simulink subsystem "WinchControl"  (R2022b)
settings: Solver=VariableStepAuto  StartTime=0.0  StopTime=10.0  RelTol=1e-3
undefined symbols (not defined in the file): constr, DiscIntNeverNeededParam, params, winchParameter
libraries: simulink x4
settings Model: Creator=dylaneijkelhof  LastModifiedBy=jesse
settings SolverCC: AlgebraicLoopSolver=TrustRegion
settings DebuggingCC: UnconnectedInputMsg=warning  UnconnectedOutputMsg=warning  UnconnectedLineMsg=warning  SFMachineParentedDataDiag=warning
settings ModelReferenceCC: EnableRefExpFcnMdlSchedulingChecks=on

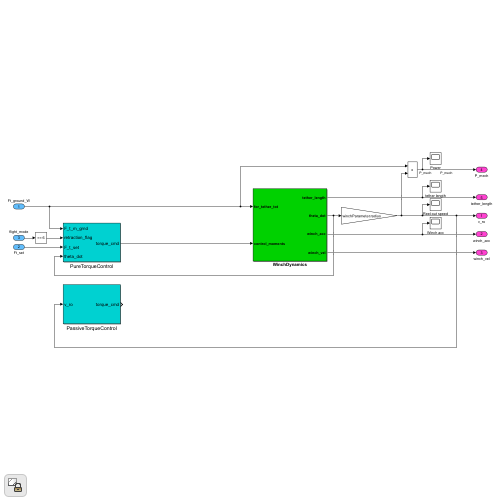
[thumbnail: Simulink's stored preview of the top-level diagram]
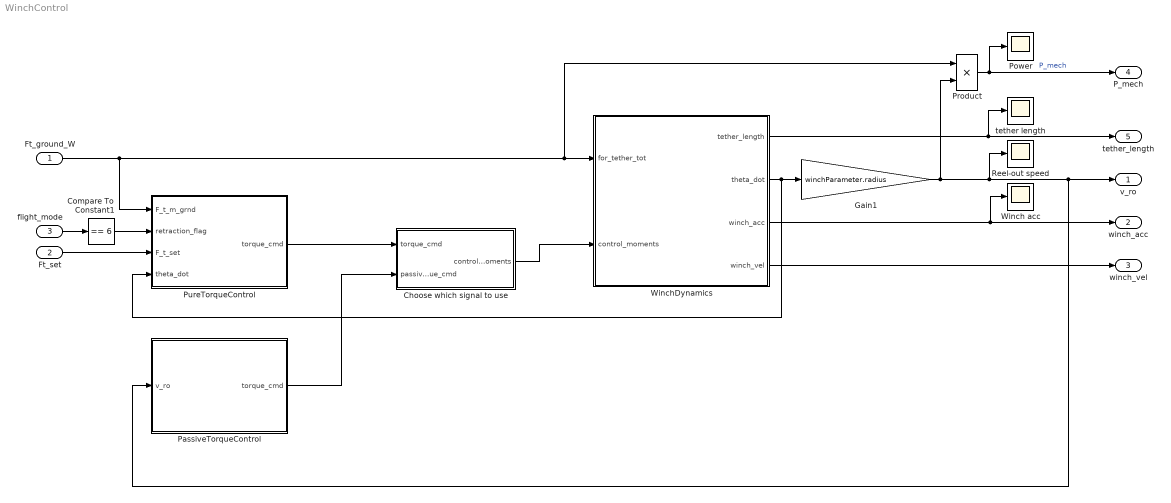
== system WinchControl ==
  Ft_ground_W : Inport  OutDataTypeStr=double  PortDimensions=1
  Ft_set : Inport  Port=2  OutDataTypeStr=double  PortDimensions=1
  flight_mode : Inport  Port=3  OutDataTypeStr=double  PortDimensions=1
  Choose which signal to use : Subsystem
  Compare To Constant1 : simulink/Logic and Bit Operations/Compare To Constant  relop===  const=6  OutDataTypeStr=boolean
  Gain1 : Gain  Gain=winchParameter.radius
  PassiveTorqueControl : Subsystem
  Power : Scope
  Product : Product
  PureTorqueControl : Subsystem
  Reel-out speed : Scope
  Winch acc : Scope
  WinchDynamics : Subsystem
  tether length : Scope
  v_ro : Outport  OutDataTypeStr=double  PortDimensions=1  VectorParamsAs1DForOutWhenUnconnected=off
  winch_acc : Outport  Port=2  OutDataTypeStr=double  PortDimensions=1  VectorParamsAs1DForOutWhenUnconnected=off
  winch_vel : Outport  Port=3  OutDataTypeStr=double  PortDimensions=1  VectorParamsAs1DForOutWhenUnconnected=off
  P_mech : Outport  Port=4  OutDataTypeStr=double  PortDimensions=1  VectorParamsAs1DForOutWhenUnconnected=off
  tether_length : Outport  Port=5  OutDataTypeStr=double  PortDimensions=1  VectorParamsAs1DForOutWhenUnconnected=off
  wires:
  Compare To Constant1/1 -> PureTorqueControl/2(retraction_flag)
  PureTorqueControl/1(torque_cmd) -> Choose which signal to use/1(torque_cmd)
  WinchDynamics/1(tether_length) -> tether length/1, tether_length/1
  WinchDynamics/3(winch_acc) -> winch_acc/1, Winch acc/1
  flight_mode/1 -> Compare To Constant1/1
  Ft_set/1 -> PureTorqueControl/3(F_t_set)
  Product/1 -> P_mech/1, Power/1  "P_mech"
  WinchDynamics/4(winch_vel) -> winch_vel/1
  Ft_ground_W/1 -> WinchDynamics/1(for_tether_tot), Product/1, PureTorqueControl/1(F_t_m_grnd)
  WinchDynamics/2(theta_dot) -> Gain1/1, PureTorqueControl/4(theta_dot)
  Gain1/1 -> v_ro/1, PassiveTorqueControl/1(v_ro), Reel-out speed/1, Product/2
  PassiveTorqueControl/1(torque_cmd) -> Choose which signal to use/2(passive_torque_cmd)
  Choose which signal to use/1(control_moments) -> WinchDynamics/2(control_moments)

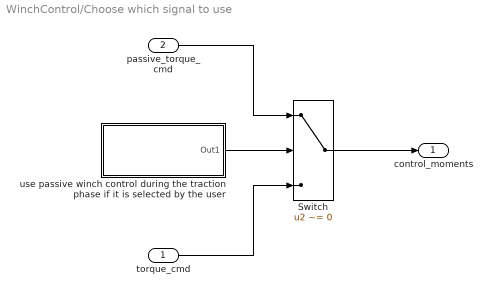
== system WinchControl/Choose which signal to use ==
  torque_cmd : Inport
  passive_torque_cmd : Inport  Port=2
  Switch : Switch  Criteria=u2 ~= 0  SaturateOnIntegerOverflow=off  InputSameDT=off
  use passive winch control during the traction phase if it is selected by the user : Subsystem
  control_moments : Outport
  wires:
  use passive winch control during the traction phase if it is selected by the user/1(Out1) -> Switch/2
  Switch/1 -> control_moments/1
  torque_cmd/1 -> Switch/3
  passive_torque_cmd/1 -> Switch/1

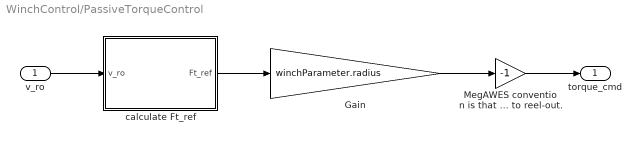
== system WinchControl/PassiveTorqueControl ==
  v_ro : Inport
  Gain : Gain  Gain=winchParameter.radius
  MegAWES convention is that a positive torque leads to reel-out. : Gain  Gain=-1
  calculate Ft_ref : MATLAB Function  TreatAsAtomicUnit=on
  torque_cmd : Outport
  wires:
  MegAWES convention is that a positive torque leads to reel-out./1 -> torque_cmd/1
  Gain/1 -> MegAWES convention is that a positive torque leads to reel-out./1
  calculate Ft_ref/1(Ft_ref) -> Gain/1
  v_ro/1 -> calculate Ft_ref/1(v_ro)

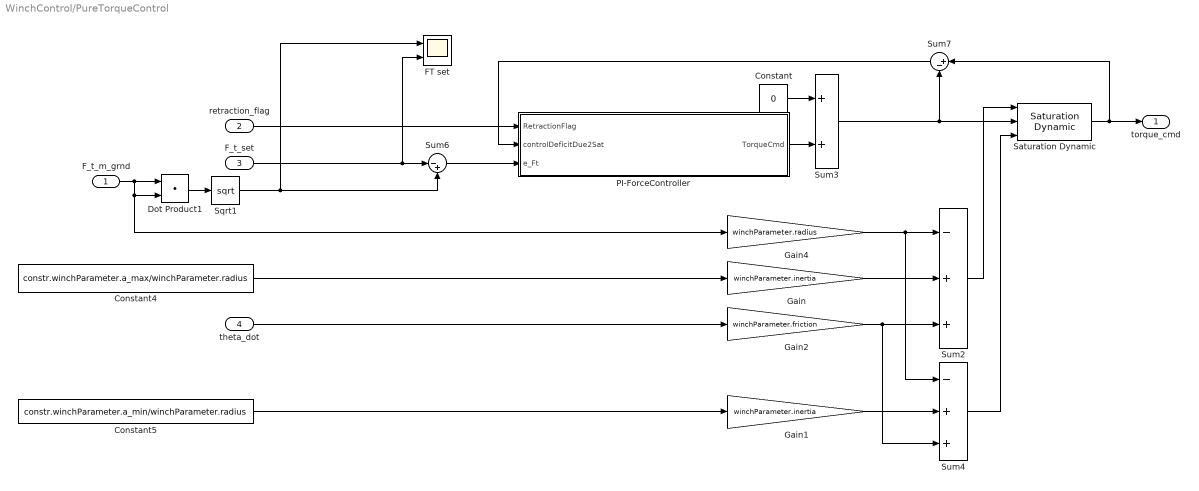
== system WinchControl/PureTorqueControl ==
  F_t_m_grnd : Inport
  retraction_flag : Inport  Port=2
  F_t_set : Inport  Port=3
  theta_dot : Inport  Port=4
  Constant : Constant  Value=0
  Constant4 : Constant  Value=constr.winchParameter.a_max/winchParameter.radius
  Constant5 : Constant  Value=constr.winchParameter.a_min/winchParameter.radius
  Dot Product1 : DotProduct  OutDataTypeStr=Inherit: Inherit via internal rule
  FT set : Scope  NumInputPorts=2
  Gain : Gain  Gain=winchParameter.inertia
  Gain1 : Gain  Gain=winchParameter.inertia
  Gain2 : Gain  Gain=winchParameter.friction
  Gain4 : Gain  Gain=winchParameter.radius
  PI-ForceController : Subsystem
  Saturation Dynamic : simulink/Discontinuities/Saturation Dynamic  OutMin=[]  OutMax=[]  OutDataTypeStr=Inherit: Same as second input  OutDataType=fixdt(1, 16)  OutScaling=2^-10  DoSatur=off
  Sqrt1 : Sqrt
  Sum2 : Sum  Inputs=-++
  Sum3 : Sum
  Sum4 : Sum  Inputs=-++
  Sum6 : Sum  Inputs=|-+
  Sum7 : Sum  Inputs=|+-
  torque_cmd : Outport  VectorParamsAs1DForOutWhenUnconnected=off
  wires:
  Saturation Dynamic/1 -> Sum7/1, torque_cmd/1
  PI-ForceController/1(TorqueCmd) -> Sum3/2
  Sum6/1 -> PI-ForceController/3(e_Ft)
  Sum7/1 -> PI-ForceController/2(controlDeficitDue2Sat)
  theta_dot/1 -> Gain2/1
  F_t_m_grnd/1 -> Gain4/1, Dot Product1/2, Dot Product1/1
  Dot Product1/1 -> Sqrt1/1
  Gain2/1 -> Sum2/3, Sum4/3
  Sum3/1 -> Sum7/2, Saturation Dynamic/2
  Sum4/1 -> Saturation Dynamic/3
  Gain1/1 -> Sum4/2
  Constant5/1 -> Gain1/1
  Sum2/1 -> Saturation Dynamic/1
  Gain/1 -> Sum2/2
  Constant4/1 -> Gain/1
  Gain4/1 -> Sum4/1, Sum2/1
  F_t_set/1 -> Sum6/1, FT set/2
  Constant/1 -> Sum3/1
  retraction_flag/1 -> PI-ForceController/1(RetractionFlag)
  Sqrt1/1 -> Sum6/2, FT set/1

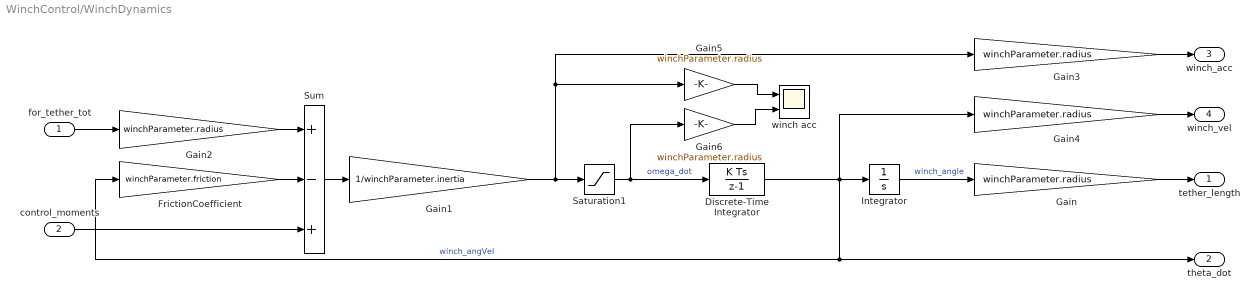
== system WinchControl/WinchDynamics ==
  for_tether_tot : Inport
  control_moments : Inport  Port=2
  Discrete-Time Integrator : DiscreteIntegrator  InitialCondition=winchParameter.lj_dot_init  SampleTime=-1  LimitOutput=on  UpperSaturationLimit=constr.winchParameter.v_max/winchParameter.radius  LowerSaturationLimit=constr.winchParameter.v_min/winchParameter.radius  ICPrevOutput=DiscIntNeverNeededParam  ICPrevScaledInput=DiscIntNeverNeededParam
  FrictionCoefficient : Gain  Gain=winchParameter.friction
  Gain{,2..6} (6 alike) : Gain  Gain=winchParameter.radius
  Gain1 : Gain  Gain=1/winchParameter.inertia
  Integrator : Integrator  InitialCondition=winchParameter.winch_angle_init
  Saturation1 : Saturate  UpperLimit=constr.winchParameter.a_max/winchParameter.radius  LowerLimit=constr.winchParameter.a_min/winchParameter.radius
  Sum : Sum  Inputs=+-+
  winch acc : Scope  NumInputPorts=2
  tether_length : Outport  VectorParamsAs1DForOutWhenUnconnected=off
  theta_dot : Outport  Port=2  VectorParamsAs1DForOutWhenUnconnected=off
  winch_acc : Outport  Port=3  VectorParamsAs1DForOutWhenUnconnected=off
  winch_vel : Outport  Port=4  VectorParamsAs1DForOutWhenUnconnected=off
  wires:
  Gain6/1 -> winch acc/2
  Gain5/1 -> winch acc/1
  Gain3/1 -> winch_acc/1
  Gain4/1 -> winch_vel/1
  Saturation1/1 -> Gain6/1, Discrete-Time Integrator/1  "omega_dot"
  Gain1/1 -> Gain3/1, Gain5/1, Saturation1/1
  for_tether_tot/1 -> Gain2/1
  FrictionCoefficient/1 -> Sum/2
  control_moments/1 -> Sum/3
  Discrete-Time Integrator/1 -> Integrator/1, Gain4/1, theta_dot/1, FrictionCoefficient/1  "winch_angVel"
  Integrator/1 -> Gain/1  "winch_angle"
  Sum/1 -> Gain1/1
  Gain2/1 -> Sum/1
  Gain/1 -> tether_length/1

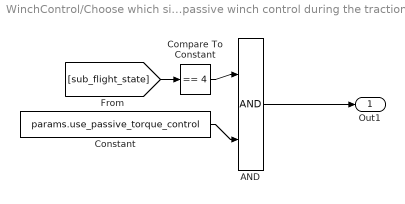
== system WinchControl/Choose which signal to use/use passive winch control during the traction phase if it is selected by the user ==
  AND : Logic  IconShape=distinctive  AllPortsSameDT=off  OutDataTypeStr=boolean
  Compare To Constant : simulink/Logic and Bit Operations/Compare To Constant  relop===  const=4  OutDataTypeStr=boolean
  Constant : Constant  Value=params.use_passive_torque_control
  Out1 : Outport
  wires:
  AND/1 -> Out1/1
  Constant/1 -> AND/2
  Compare To Constant/1 -> AND/1
  [sub_flight_state] -> Compare To Constant/1

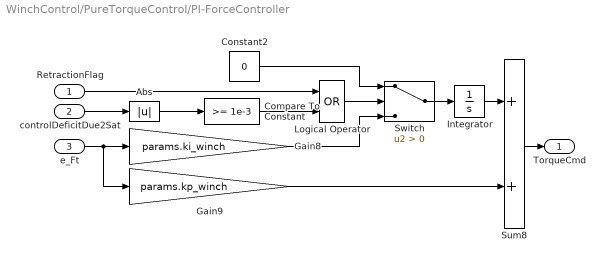
== system WinchControl/PureTorqueControl/PI-ForceController ==
  RetractionFlag : Inport
  controlDeficitDue2Sat : Inport  Port=2
  e_Ft : Inport  Port=3
  Abs : Abs  SaturateOnIntegerOverflow=off
  Compare To Constant : simulink/Logic and Bit Operations/Compare To Constant  relop=>=  const=1e-3  OutDataTypeStr=boolean
  Constant2 : Constant  Value=0
  Gain8 : Gain  Gain=params.ki_winch
  Gain9 : Gain  Gain=params.kp_winch
  Integrator : Integrator
  Logical Operator : Logic  Operator=OR  AllPortsSameDT=off  OutDataTypeStr=boolean
  Sum8 : Sum
  Switch : Switch  Criteria=u2 > Threshold  SaturateOnIntegerOverflow=off  InputSameDT=off
  TorqueCmd : Outport  VectorParamsAs1DForOutWhenUnconnected=off
  wires:
  Logical Operator/1 -> Switch/2
  RetractionFlag/1 -> Logical Operator/1
  controlDeficitDue2Sat/1 -> Abs/1
  e_Ft/1 -> Gain9/1, Gain8/1
  Abs/1 -> Compare To Constant/1
  Integrator/1 -> Sum8/1
  Compare To Constant/1 -> Logical Operator/2
  Gain8/1 -> Switch/3
  Gain9/1 -> Sum8/2
  Constant2/1 -> Switch/1
  Switch/1 -> Integrator/1
  Sum8/1 -> TorqueCmd/1

== matlab function WinchControl/PassiveTorqueControl/calculate Ft_ref ==
  data: v_ro input; Ft_ref output; winchParameter parameter; params parameter
function Ft_ref = fcn(v_ro, winchParameter, params)
% From Zgraggen (2016): "Automatic Retraction and Full-Cycle Operation for a
% Class of Airborne Wind Energy Generators".

C = 7.7008e3;  % Hard-coded for the MegAWES kite.
r_m = winchParameter.radius;

if v_ro > 0
    Ft_ref = 4*C*v_ro^2;
else
    Ft_ref = 0.0;
end

% If the winch controls the max tether force, implement a ceiling. + There
% is always a minimum tether force.
winch_controls_max_tether_force = ~(params.kite_alpha_mode == 3);
if winch_controls_max_tether_force
    Ft_ref = min(max(Ft_ref, params.winch_Ft_min), params.winch_Ft_max);
else
    Ft_ref = max(Ft_ref, params.winch_Ft_min);
end
